simulink model "TrqLimit"  (R2019b)
settings: Solver=VariableStepAuto  StartTime=0.0  StopTime=10.0  RelTol=1e-3
values from neighbouring files (symbols this model uses):
  RearRatio = 0.8    [VehCtrlMdelDictionary.sldd]
libraries: simulink x6
settings Model: Creator=12045  LastModifiedBy=12045
settings OptimizationCC: DefaultParameterBehavior=Inlined  EnhancedBackFolding=on  PassReuseOutputArgsAs=Individual arguments  ZeroExternalMemoryAtStartup=off  ZeroInternalMemoryAtStartup=off  OptimizeBlockOrder=speed  DifferentSizesBufferReuse=on  OptimizationCustomize=off  EfficientTunableParamExpr=on
settings DebuggingCC: ParameterTunabilityLossMsg=error
settings SFSimCC: MATLABDynamicMemAlloc=off
settings RTWCC: Description=AUTOSAR  SystemTargetFile=autosar.tlc  GenCodeOnly=on  TemplateMakefile=ert_default_tmf  GenerateReport=on  IncludeHyperlinkInReport=on  LaunchReport=on  GenerateTraceInfo=on  GenerateTraceReport=on  GenerateTraceReportSl=on  GenerateTraceReportSf=on  GenerateTraceReportEml=on
settings CodeAppCC: ForceParamTrailComments=on  IgnoreCustomStorageClasses=off  OperatorAnnotations=on  SimulinkDataObjDesc=on  SFDataObjDesc=on  InsertBlockDesc=on
settings STFCustomTargetCC: TargetLangStandard=C99 (ISO)  MultiwordLength=256  ParMdlRefBuildCompliant=on  CompOptLevelCompliant=on  IncludeMdlTerminateFcn=off  CombineOutputUpdateFcns=on  SuppressErrorStatus=on  ERTCustomFileBanners=on  SupportNonFinite=off  SupportComplex=off  SupportContinuousTime=off  SupportNonInlinedSFcns=off  RemoveResetFunc=on  MATLABClassNameForMDSCustomization=Simulink.SoftwareTarget.ERTCustomization  AutosarCompliant=on  UseToolchainInfoCompliant=on  LookupTableObjectStructAxisOrder=2,1,3,4,...  LUTObjectStructOrderEvenSpacing=Size,Table,Breakpoints  SystemTargetFile=autosar.tlc
settings ERTTargetCC: TargetLangStandard=C99 (ISO)  ConcurrentExecutionCompliant=off  IncludeMdlTerminateFcn=off  SuppressErrorStatus=on  SupportNonFinite=off  SupportComplex=off  ModelStepFunctionPrototypeControlCompliant=off  CPPClassGenCompliant=off  AutosarCompliant=on  LookupTableObjectStructAxisOrder=2,1,3,4,...  LUTObjectStructOrderEvenSpacing=Size,Table,Breakpoints  InlinedParameterPlacement=NonHierarchical  ERTCustomFileTemplate=example_file_process.tlc

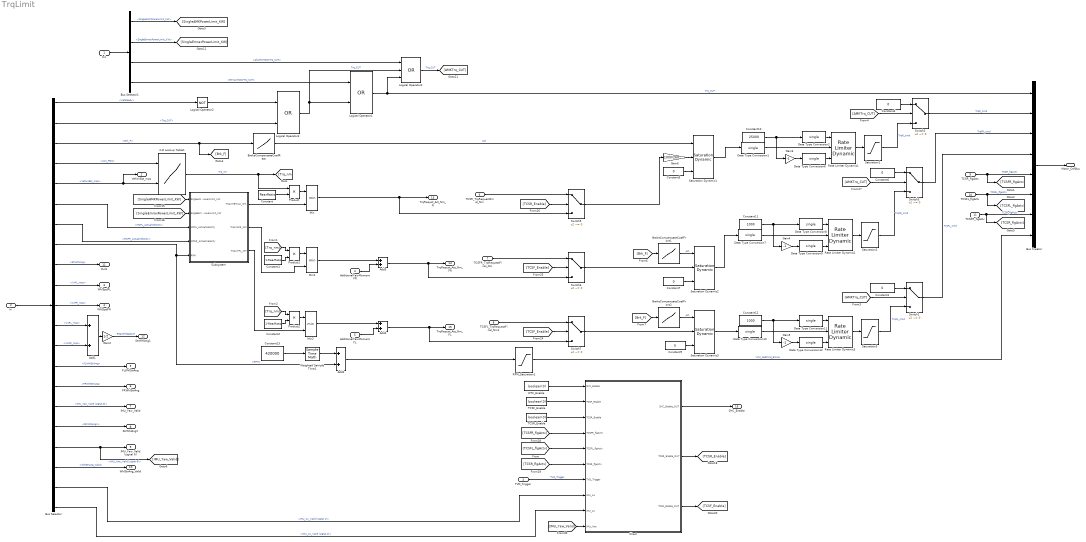
== system TrqLimit ==
  In1 : Inport
  In : Inport  Port=2
  TVD_Trigger : Inport  Port=3
  AdditionalYawMomentFR : Inport  Port=4
  AdditionalYawMomentFL : Inport  Port=5
  TCSR_TrqRequestFinal_Nm : Inport  Port=6
  TCSFR_TrqRequestFinal_Nm : Inport  Port=7
  TCSFL_TrqRequestFinal_Nm1 : Inport  Port=8
  TCSR_flgActv : Inport  Port=9
  TCSFL_flgActv : Inport  Port=10
  TCSFR_flgActv : Inport  Port=11
  2-D Lookup Table1 : Lookup_n-D  BreakpointsForDimension1=single([0 10 20 30 40 50 60 70 80 90 100])  BreakpointsForDimension2=single([5.40000009536743 10.8000001907349 16.2000007629395 21.6000003814697 27 32.4000015258789 37.7999992370605 43.2000007629395 48.5999984741211 54 59.4000015258789 64.8000030517578 70.1999969482422 75.5999984741211 81 86.4000015258789 91.8000030517578 97.1999969482422 102.599998474121 108])  BreakpointsForDimension1DataTypeStr=single  BreakpointsForDimension2DataTypeStr=single  Table=single([0 0 0 0 0 0 0 0 0 0 0 0 0 0 0 0 0 0 0 0;20 20 20 20 20 20 20 18 18 18 17 17 16 16 15 15 15 14 14 14;35 35 35 35 35 35 30 30 25 25 25 25 20 20 20 20 20 20 20 18;50 50 50 50 50 50 50 50 50 40 40 40 40 40 40 40 40 40 38 35;79 79 79 79 85 85 85 90 95 100 110 110 110 100 90 90 80 72 70 65;100 100 100 105 105 105 110 110 110 110 115 115 125 125 120 110 90 80 76 70;120 120 120 120 125 125 125 135 135 135 135 135 135 130 130 120 100 90 82 74;125 125 125 130 135 140 145 155 155 155 155 155 155 155 155 135 110 100 88 82;130 160 160 160 160 170 160 160 160 160 160 160 160 160 160 142 120 105 94 88;130 160 160 160 160 170 160 160 160 160 160 160 160 160 160 142 120 105 95 91;170 170 180 180 180 210 200 200 200 200 200 200 190 180 180 152 133 118 106 100])  InternalRulePriority=Speed  RndMeth=Simplest  InputSameDT=on
  Add{1..4} (4 alike) : Sum
  BrakeCompensateCoefFront1 : Lookup_n-D  NumberOfTableDimensions=1  BreakpointsForDimension1=single([550,2000]);  Table=single([20,0]);  ExtrapMethod=Clip  InternalRulePriority=Speed  OutDataTypeStr=single  RndMeth=Simplest  InputSameDT=on
  BrakeCompensateCoefFront2 : Lookup_n-D  NumberOfTableDimensions=1  BreakpointsForDimension1=single([550,2000]);  Table=single([20,0]);  ExtrapMethod=Clip  InternalRulePriority=Speed  OutDataTypeStr=single  RndMeth=Simplest  InputSameDT=on
  BrakeCompensateCoefRear : Lookup_n-D  NumberOfTableDimensions=1  BreakpointsForDimension1=single([550,2000]);  Table=single([1000,0]);  ExtrapMethod=Clip  InternalRulePriority=Speed  OutDataTypeStr=single  RndMeth=Simplest  InputSameDT=on
  Bus Creator : BusCreator  Inputs=8
  Bus Selector : BusSelector  OutputSignals=VehReady,VCUReceive.signal1.AccBrkPedal_Processing.Trq_CUT,VCUReceive.signal1.AccBrkPedal_Processing.Brk_F,VCUReceive.signal1.AccBrkPedal_Processing.Acc_POS,VCUReceive.VehVxEst_mps,VCUReceive.signal1.BUS.AMKMCUtoVCU_BUS.FLAMKMCUtoVCU1.MCFL_ActualVelocity,VCUReceive.signal1.BUS.AMKMCUtoVCU_BUS.FRAMKMCUtoVCU1.MCFR_ActualVelocity,VCUReceive.signal1.BUS.EMRAXMCU_Receive.MCU_state.RPM,VCUReceive.signal1.SWAS_Processing.StrWhlAng,VCUReceive.Vxii_mps.VxFL_mps,VCUReceive.Vxii_mps.VxFR_mps,VCUReceive.Vxii_mps.VxRL_mps,VCUReceive.Vxii_mps.VxRR_mps,VCUReceive.signal1.SWAS_Processing.FLWhlStrAng,VCUReceive.signal1.SWAS_Processing.FRWhlStrAng,VCUReceive.signal1.IMU_Processing.IMU_Yaw_Valid (signal 3),VCUReceive.signal1.SWAS_Processing.StrWhlAngV,VCUReceive.signal1.IMU_Processing.IMU_Yaw_Valid (signal 6),VCUReceive.signal1.SWAS_Processing.WhlStrAng_Valid,VCUReceive.signal1.IMU_Processing.IMU_Ax_Valid (signal 1),VCUReceive.signal1.IMU_Processing.IMU_Ay_Valid (signal 2)
  Bus Selector1 : BusSelector  OutputSignals=SingleAMKPowerLimit_KW,SingleEmraxPowerLimit_KW,allAMKMotorTrq_CUT,EmraxMotorTrq_CUT
  Chart : Stateflow chart  TreatAsAtomicUnit=on
  Constant : Constant  Value=RearRatio
  Constant1 : Constant  Value=1-RearRatio
  Constant10 : Constant  Value=25000  OutDataTypeStr=single
  Constant11 : Constant  Value=1000  OutDataTypeStr=single
  Constant12 : Constant  Value=1000  OutDataTypeStr=single
  Constant13 : Constant  Value=420000  OutDataTypeStr=single
  Constant2 : Constant  Value=1-RearRatio
  Constant{3..7,9} (6 alike) : Constant  Value=0  OutDataTypeStr=single
  DTC_Enable : Constant  Value=boolean(0)
  Data Type Conversion{1..2,6..12} (9 alike) : DataTypeConversion  OutDataTypeStr=single
  Gain2 : Gain  Gain=1/2
  Gain3 : Gain  Gain=-1
  Gain4 : Gain  Gain=-1
  Gain5 : Gain  Gain=-1
  Gain6 : Gain  Gain=1000/260
  Logical Operator1 : Logic  Operator=OR  AllPortsSameDT=off  OutDataTypeStr=boolean
  Logical Operator2 : Logic  Operator=NOT  AllPortsSameDT=off  OutDataTypeStr=boolean
  Logical Operator3 : Logic  Operator=OR  AllPortsSameDT=off  OutDataTypeStr=boolean
  Logical Operator4 : Logic  Operator=OR  Inputs=3  AllPortsSameDT=off  OutDataTypeStr=boolean
  Min : MinMax  Inputs=2
  Min1 : MinMax  Inputs=2
  Min2 : MinMax  Inputs=2
  Product : Product
  Product1 : Product
  Product2 : Product
  RPM_Saturation1 : Saturate  UpperLimit=5000  LowerLimit=-50
  Rate Limiter Dynamic1 : simulink/Discontinuities/Rate Limiter Dynamic
      settings: SourceProductName=Simulink
  Rate Limiter Dynamic2 : simulink/Discontinuities/Rate Limiter Dynamic
      settings: SourceProductName=Simulink
  Rate Limiter Dynamic3 : simulink/Discontinuities/Rate Limiter Dynamic
      settings: SourceProductName=Simulink
  Saturation Dynamic1 : simulink/Discontinuities/Saturation Dynamic  OutMin=[]  OutMax=[]  OutDataTypeStr=single  OutputDataTypeScalingMode=single  OutDataType=fixdt(1, 16)  OutScaling=2^-10  DoSatur=off
  Saturation Dynamic2 : simulink/Discontinuities/Saturation Dynamic  OutMin=[]  OutMax=[]  OutDataTypeStr=single  OutputDataTypeScalingMode=single  OutDataType=fixdt(1, 16)  OutScaling=2^-10  DoSatur=off
  Saturation Dynamic3 : simulink/Discontinuities/Saturation Dynamic  OutMin=[]  OutMax=[]  OutDataTypeStr=single  OutputDataTypeScalingMode=single  OutDataType=fixdt(1, 16)  OutScaling=2^-10  DoSatur=off
  Saturation1 : Saturate  UpperLimit=1000  LowerLimit=0
  Saturation2 : Saturate  UpperLimit=20  LowerLimit=0
  Saturation3 : Saturate  UpperLimit=20  LowerLimit=0
  Subsystem : Subsystem
  Switch{1..3,5..7} (6 alike) : Switch  Criteria=u2 ~= 0
  TCSF_Enable : Constant  Value=boolean(0)  OutDataTypeStr=boolean
  TCSR_Enable : Constant  Value=boolean(0)  OutDataTypeStr=boolean
  Weighted Sample Time1 : SampleTimeMath  TsampMathOp=*
  Motor_CtrlBus : Outport  VectorParamsAs1DForOutWhenUnconnected=off
  VehVxEst_mps : Outport  Port=2
  WhlSpdFL : Outport  Port=3
  WhlSpdFR : Outport  Port=4
  FLWhlStrAng : Outport  Port=5
  FRWhlStrAng : Outport  Port=6
  IMU_Yaw_Valid : Outport  Port=7
  StrWhlAngV : Outport  Port=8
  IMU_Yaw_Valid (signal 6) : Outport  Port=9
  WhlStrAng_Valid : Outport  Port=10
  Out1 : Outport  Port=11
  StrWhlAng1 : Outport  Port=12
  TrqRequst_Act_Nm_R : Outport  Port=13
  TrqRequst_Act_Nm_FR : Outport  Port=14
  TrqRequst_Act_Nm_FL : Outport  Port=15
  DYC_Enable : Outport  Port=16
  wires:
  Data Type Conversion6/1 -> Rate Limiter Dynamic1/3
  Bus Selector/11 -> WhlSpdFR/1  "<VxFR_mps>"
  Saturation Dynamic2/1 -> Data Type Conversion7/1
  Constant10/1 -> Gain3/1, Data Type Conversion2/1
  Gain3/1 -> Data Type Conversion6/1
  Rate Limiter Dynamic2/1 -> Saturation2/1
  TCSFR_flgActv/1 -> [TCSR_flgActv], Bus Creator/7  "TCSR_flgActv"
  TCSR_flgActv/1 -> [TCSFR_flgActv], Bus Creator/5  "TCSR_flgActv"
  TCSFL_TrqRequestFinal_Nm1/1 -> Switch7/1
  Bus Selector/6 -> Subsystem/3(MCFL_ActualVelocity)  "<MCFL_ActualVelocity>"
  BrakeCompensateCoefFront2/1 -> Saturation Dynamic3/1  "pct"
  [Brk_F] -> BrakeCompensateCoefFront2/1
  Bus Selector/4 -> 2-D Lookup Table1/1  "<Acc_POS>"
  Bus Selector/9 -> Out1/1  "<StrWhlAng>"
  Constant7/1 -> Saturation Dynamic2/3
  [Trq_nm] -> Product2/1
  2-D Lookup Table1/1 -> Product/1, [Trq_nm]  "Trq_nm"
  TCSFR_TrqRequestFinal_Nm/1 -> Switch6/1
  Constant6/1 -> Switch3/1
  Subsystem/2(TrqLimFR_Nm) -> Min1/2
  Saturation Dynamic1/1 -> Data Type Conversion1/1
  Bus Selector/5 -> VehVxEst_mps/1, 2-D Lookup Table1/2  "<VehVxEst_mps>"
  Logical Operator2/1 -> Logical Operator3/1
  Logical Operator1/1 -> Bus Creator/1, Logical Operator4/3  "Trq_CUT"
  Bus Selector/2 -> Logical Operator3/2  "<Trq_CUT>"
  In/1 -> Bus Selector/1
  Chart/3(TCSF_Enable_OUT) -> [TCSF_Enable]
  Bus Selector/10 -> WhlSpdFL/1  "<VxFL_mps>"
  [IMU_Yaw_Valid] -> Chart/10(IMU_Yaw)
  Data Type Conversion12/1 -> Rate Limiter Dynamic3/3
  Switch3/1 -> Bus Creator/3  "TrqFR_cmd"
  [SingleEmraxPowerLimit_KW] -> Subsystem/2(SingleEmraxPowerLimit_KW)
  Bus Selector/18 -> IMU_Yaw_Valid (signal 6)/1, [IMU_Yaw_Valid]  "<IMU_Yaw_Valid (signal 6)>"
  TCSF_Enable/1 -> Chart/2(TCSF_Enable)
  Logical Operator4/1 -> [AMKTrq_CUT]  "Trq_CUT"
  Bus Selector/13 -> Add1/2  "<VxRR_mps>"
  Bus Selector1/1 -> [SingleAMKPowerLimit_KW]  "<SingleAMKPowerLimit_KW>"
  Add3/1 -> TrqRequst_Act_Nm_FR/1, Switch6/3
  Bus Selector/20 -> Chart/8(IMU_Ax)  "<IMU_Ax_Valid (signal 1)>"
  [TCSFR_flgActv] -> Chart/4(TCSFR_flgActv)
  Saturation Dynamic3/1 -> Data Type Conversion10/1
  Bus Selector/21 -> Chart/9(IMU_Ay)  "<IMU_Ay_Valid (signal 2)>"
  Chart/1(DYC_Enable_OUT) -> DYC_Enable/1
  TVD_Trigger/1 -> Chart/7(TVD_Trigger)  "TVD_Trigger"
  Bus Creator/1 -> Motor_CtrlBus/1
  Bus Selector/17 -> StrWhlAngV/1  "<StrWhlAngV>"
  [TCSR_flgActv] -> Chart/6(TCSR_flgActv)
  Chart/2(TCSR_Enable_OUT) -> [TCSR_Enable]
  [AMKTrq_CUT] -> Switch3/2
  Constant1/1 -> Product1/2
  [TCSFL_flgActv] -> Chart/5(TCSFL_flgActv)
  Constant9/1 -> Saturation Dynamic3/3
  DTC_Enable/1 -> Chart/1(DYC_Enable)
  [Trq_nm] -> Product1/1
  TCSR_Enable/1 -> Chart/3(TCSR_Enable)
  Bus Selector/16 -> IMU_Yaw_Valid/1  "<IMU_Yaw_Valid (signal 3)>"
  Gain6/1 -> Saturation Dynamic1/2
  Min1/1 -> Add3/1
  Bus Selector/19 -> WhlStrAng_Valid/1  "<WhlStrAng_Valid>"
  Logical Operator3/1 -> Logical Operator4/2, Logical Operator1/2  "Trq_CUT"
  Bus Selector/15 -> FRWhlStrAng/1  "<FRWhlStrAng>"
  Constant/1 -> Product/2
  Bus Selector/12 -> Add1/1  "<VxRL_mps>"
  Constant2/1 -> Product2/2
  Bus Selector1/2 -> [SingleEmraxPowerLimit_KW]  "<SingleEmraxPowerLimit_KW>"
  BrakeCompensateCoefRear/1 -> Saturation Dynamic1/1  "pct"
  Bus Selector/3 -> [Brk_F], BrakeCompensateCoefRear/1  "<Brk_F>"
  Product/1 -> Min/1
  AdditionalYawMomentFR/1 -> Add3/2
  Bus Selector1/3 -> Logical Operator4/1  "<allAMKMotorTrq_CUT>"
  RPM_Saturation1/1 -> Bus Creator/8  "VCU_SpdCmd_Emrax"
  Constant5/1 -> Saturation Dynamic1/3
  Data Type Conversion1/1 -> Rate Limiter Dynamic1/2
  Product1/1 -> Min1/1
  Bus Selector1/4 -> Logical Operator1/1  "<EmraxMotorTrq_CUT>"
  Subsystem/1(TrqLimEmrax_Nm) -> Min/2
  Bus Selector/1 -> Logical Operator2/1  "<VehReady>"
  [TCSF_Enable] -> Switch7/2
  Switch7/1 -> Saturation Dynamic3/2
  Add4/1 -> TrqRequst_Act_Nm_FL/1, Switch7/3
  Gain2/1 -> StrWhlAng1/1  "RearWhlSpdAve"
  TCSR_TrqRequestFinal_Nm/1 -> Switch5/1
  Rate Limiter Dynamic3/1 -> Saturation3/1
  Weighted Sample Time1/1 -> Add2/1
  [TCSR_Enable] -> Switch5/2
  Add1/1 -> Gain2/1
  Switch2/1 -> Bus Creator/2  "TrqR_cmd"
  Data Type Conversion10/1 -> Rate Limiter Dynamic3/2
  Min2/1 -> Add4/1
  Add2/1 -> RPM_Saturation1/1
  [SingleAMKPowerLimit_KW] -> Subsystem/1(SingleAMKPowerLimit_KW)
  [TCSF_Enable] -> Switch6/2
  Product2/1 -> Min2/1
  BrakeCompensateCoefFront1/1 -> Saturation Dynamic2/1  "pct"
  Gain4/1 -> Data Type Conversion9/1
  Data Type Conversion8/1 -> Rate Limiter Dynamic2/1
  Gain5/1 -> Data Type Conversion12/1
  Switch5/1 -> Gain6/1
  Constant11/1 -> Data Type Conversion8/1, Gain4/1
  Switch1/1 -> Bus Creator/4  "TrqFL_cmd"
  In1/1 -> Bus Selector1/1
  Bus Selector/8 -> Subsystem/5(RPM), Add2/2  "<RPM>"
  Data Type Conversion7/1 -> Rate Limiter Dynamic2/2
  Rate Limiter Dynamic1/1 -> Saturation1/1
  AdditionalYawMomentFL/1 -> Add4/2
  Min/1 -> TrqRequst_Act_Nm_R/1, Switch5/3
  Bus Selector/7 -> Subsystem/4(MCFR_ActualVelocity)  "<MCFR_ActualVelocity>"
  Bus Selector/14 -> FLWhlStrAng/1  "<FLWhlStrAng>"
  Data Type Conversion2/1 -> Rate Limiter Dynamic1/1
  Switch6/1 -> Saturation Dynamic2/2
  Subsystem/3(TrqLimFL_Nm) -> Min2/2
  Data Type Conversion11/1 -> Rate Limiter Dynamic3/1
  Data Type Conversion9/1 -> Rate Limiter Dynamic2/3
  Constant13/1 -> Weighted Sample Time1/1
  [Brk_F] -> BrakeCompensateCoefFront1/1
  Constant12/1 -> Gain5/1, Data Type Conversion11/1
  TCSFL_flgActv/1 -> [TCSFL_flgActv], Bus Creator/6  "TCSFL_flgActv"
  Saturation2/1 -> Switch3/3  "TrqFR_cmd"
  [AMKTrq_CUT] -> Switch1/2
  Constant3/1 -> Switch1/1
  Saturation3/1 -> Switch1/3  "TrqFL_cmd"
  [AMKTrq_CUT] -> Switch2/2
  Constant4/1 -> Switch2/1
  Saturation1/1 -> Switch2/3  "TrqR_cmd"

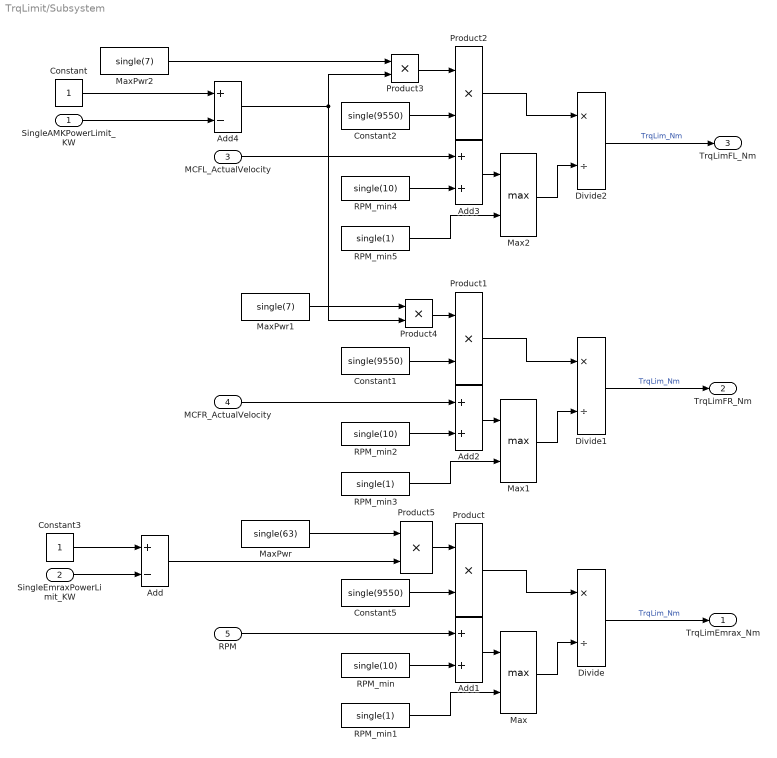
== system TrqLimit/Subsystem ==
  SingleAMKPowerLimit_KW : Inport
  SingleEmraxPowerLimit_KW : Inport  Port=2
  MCFL_ActualVelocity : Inport  Port=3
  MCFR_ActualVelocity : Inport  Port=4
  RPM : Inport  Port=5
  Add : Sum  Inputs=+-
  Add1 : Sum
  Add2 : Sum
  Add3 : Sum
  Add4 : Sum  Inputs=+-
  Constant : Constant
  Constant1 : Constant  Value=single(9550)  OutDataTypeStr=single
  Constant2 : Constant  Value=single(9550)  OutDataTypeStr=single
  Constant3 : Constant
  Constant5 : Constant  Value=single(9550)  OutDataTypeStr=single
  Divide : Product  Inputs=*/
  Divide1 : Product  Inputs=*/
  Divide2 : Product  Inputs=*/
  Max : MinMax  Function=max  Inputs=2
  Max1 : MinMax  Function=max  Inputs=2
  Max2 : MinMax  Function=max  Inputs=2
  MaxPwr : Constant  Value=single(63)  OutDataTypeStr=single
  MaxPwr1 : Constant  Value=single(7)  OutDataTypeStr=single
  MaxPwr2 : Constant  Value=single(7)  OutDataTypeStr=single
  Product{,1..5} (6 alike) : Product
  RPM_min : Constant  Value=single(10)  OutDataTypeStr=single
  RPM_min1 : Constant  Value=single(1)  OutDataTypeStr=single
  RPM_min2 : Constant  Value=single(10)  OutDataTypeStr=single
  RPM_min3 : Constant  Value=single(1)  OutDataTypeStr=single
  RPM_min4 : Constant  Value=single(10)  OutDataTypeStr=single
  RPM_min5 : Constant  Value=single(1)  OutDataTypeStr=single
  TrqLimEmrax_Nm : Outport
  TrqLimFR_Nm : Outport  Port=2
  TrqLimFL_Nm : Outport  Port=3
  wires:
  Max/1 -> Divide/2
  Divide/1 -> TrqLimEmrax_Nm/1  "TrqLim_Nm"
  RPM_min1/1 -> Max/2
  Constant5/1 -> Product/2
  RPM/1 -> Add1/1
  Product/1 -> Divide/1
  RPM_min/1 -> Add1/2
  Add1/1 -> Max/1
  Add2/1 -> Max1/1
  RPM_min2/1 -> Add2/2
  MaxPwr1/1 -> Product4/1
  Product1/1 -> Divide1/1
  MCFR_ActualVelocity/1 -> Add2/1
  Constant1/1 -> Product1/2
  RPM_min3/1 -> Max1/2
  Divide1/1 -> TrqLimFR_Nm/1  "TrqLim_Nm"
  Max1/1 -> Divide1/2
  Max2/1 -> Divide2/2
  Divide2/1 -> TrqLimFL_Nm/1  "TrqLim_Nm"
  RPM_min5/1 -> Max2/2
  Constant2/1 -> Product2/2
  MCFL_ActualVelocity/1 -> Add3/1
  Product2/1 -> Divide2/1
  RPM_min4/1 -> Add3/2
  Add3/1 -> Max2/1
  MaxPwr/1 -> Product5/1
  Add/1 -> Product5/2
  Product5/1 -> Product/1
  Product3/1 -> Product2/1
  Add4/1 -> Product3/2, Product4/2
  Product4/1 -> Product1/1
  Constant/1 -> Add4/1
  MaxPwr2/1 -> Product3/1
  SingleAMKPowerLimit_KW/1 -> Add4/2
  SingleEmraxPowerLimit_KW/1 -> Add/2
  Constant3/1 -> Add/1

== stateflow chart TrqLimit/Chart ==
  state A
    en:
    if abs(IMU_Ay)>0.5
    a=atan(IMU_Ax/IMU_Ay)*180/pi;
    else
    a = 0;
    end
    b=sqrt(power(IMU_Ax,2)+power(IMU_Ay,2));
  state InitState
  state DYC_Disenable
    en:
    DYC_Enable_OUT=0;
    DYC_flag=0;
  state TCSR_Disenable
    en:
    TCSR_Enable_OUT=0;
  state TCSR_Enable
    en:
    TCSR_Enable_OUT=1;
  state TCSF_Disenable
    en:
    TCSF_Enable_OUT=0;
  state TCSF_Enable
    en:
    TCSF_Enable_OUT=1;
  state DYC_Enable
    en:
    DYC_Enable_OUT=1;
    DYC_flag=1;
  state B
    en:
    TCSR_Enable_OUT=1;
  state F_TVD_TCS_STATE
  state C
    en:
    TCSR_Enable_OUT=0;
  (default) -> InitState [order 1]
  (default) -> A [order 2]
  A -> A
  InitState -> TCSR_Disenable [order 5] : [~TCSR_Enable]
  InitState -> TCSR_Enable [order 6] : [TCSR_Enable]
  TCSF_Disenable -> InitState : [TCSF_Enable]
  InitState -> TCSF_Disenable [order 4] : [~TCSF_Enable]
  InitState -> TCSF_Enable [order 3] : [TCSF_Enable&&DYC_flag&&~DYC_flag&&a>60&&a<-60&&IMU_Ax>2&&b<5&&IMU_Yaw<50]
  TCSF_Enable -> InitState : [b>5]
  DYC_Disenable -> InitState : [DYC_Enable]
  InitState -> DYC_Disenable [order 2] : [~DYC_Enable]
  DYC_Enable -> InitState : [IMU_Yaw>=50||IMU_Ay>=5||b>=5]
  InitState -> DYC_Enable [order 1] : [DYC_Enable&&IMU_Yaw<=50&&IMU_Ay<5&&b<5]
  TCSR_Disenable -> TCSR_Enable : [TCSR_Enable]
  TCSR_Enable -> TCSR_Disenable : [~TCSR_Enable]
  F_TVD_TCS_STATE -> B [order 1] : [DYC_flag&&IMU_Yaw<=30&&a>=30&&a<=-30&&b<=3]
  B -> F_TVD_TCS_STATE : [~DYC_flag||IMU_Yaw>30||a>30||a>-30||b>3]
  (default) -> F_TVD_TCS_STATE [order 3]
  C -> F_TVD_TCS_STATE : [DYC_flag&&IMU_Yaw<=30&&a>=30&&a<=-30&&b<=3]
  F_TVD_TCS_STATE -> C [order 2] : [~DYC_flag||IMU_Yaw>30||a>30||a>-30||b>3]
  data: DYC_Enable input; TCSF_Enable input; TCSR_Enable input; TCSFR_flgActv input; TCSFL_flgActv input; TCSR_flgActv input; TVD_Trigger input; DYC_Enable_OUT output; TCSR_Enable_OUT output; TCSF_Enable_OUT output; IMU_Ax input; IMU_Ay input; IMU_Yaw input; a local; b local; DYC_flag local
